simulink model "Sim_Metabolico_ParamE2"  (R2024b)
settings: Solver=ode15s  StartTime=0.0  StopTime=30  RelTol=1e-12  AbsTol=1e-6  EnableMultiTasking=on
values from neighbouring files (symbols this model uses):
  k_I_sec = 10    [Fig10_ParametricAnalysis_kIsec_JTB.m]    (also in Fig11_ParametricAnalysis_kIupJTB.m; Fig12_ParametricAnalysis_kP4sec_JTB.m; SensitivityAnalysisFIM_JTBpaper.m)
  k_I_up = 12    [Fig10_ParametricAnalysis_kIsec_JTB.m]    (also in Fig11_ParametricAnalysis_kIupJTB.m; Fig12_ParametricAnalysis_kP4sec_JTB.m; SensitivityAnalysisFIM_JTBpaper.m = 11.999988)
settings Model: Creator=Usuario  LastModifiedBy=carolinaramirezmazo
settings SolverCC: AutoScaleAbsTol=off  AlgebraicLoopSolver=TrustRegion
settings DataIOCC: LimitDataPoints=on  SaveFormat=Array  ReturnWorkspaceOutputs=off
settings OptimizationCC: LifeSpan=inf
settings DebuggingCC: SolverPrmCheckMsg=warning  UnconnectedInputMsg=warning  UnconnectedOutputMsg=warning  UnconnectedLineMsg=warning  SFUnexpectedBacktrackingDiag=warning  SFNoUnconditionalDefaultTransitionDiag=warning  SFExecutionAtInitializationDiag=none  ArithmeticOperatorsInVariantConditions=warning
settings HardwareCC: ProdBitPerPointer=32  ProdBitPerSizeT=32  ProdBitPerPtrDiffT=32  ProdLargestAtomicFloat=None  ProdIntDivRoundTo=Undefined  ProdEndianess=Unspecified  ProdWordSize=32  ProdHWDeviceType=32-bit Generic
settings ModelReferenceCC: EnableRefExpFcnMdlSchedulingChecks=on  PropagateSignalLabelsOutOfModel=off
settings SFSimCC: SimUseLocalCustomCode=off  CustomCodeUndefinedFunction=UseInterfaceOnly
settings RTWCC: RTWUseLocalCustomCode=off  GPUComputeCapability=3.5  DLArmComputeVersion=19.05
settings CodeAppCC: StateflowObjectComments=on
settings GRTTargetCC: TargetLangStandard=C89/C90 (ANSI)
settings ConfigComp: CovMetricSettings=dw  CovSaveCumulativeToWorkspaceVar=on  CovSaveSingleToWorkspaceVar=on  CovExternalEMLEnable=off  CovSFcnEnable=off

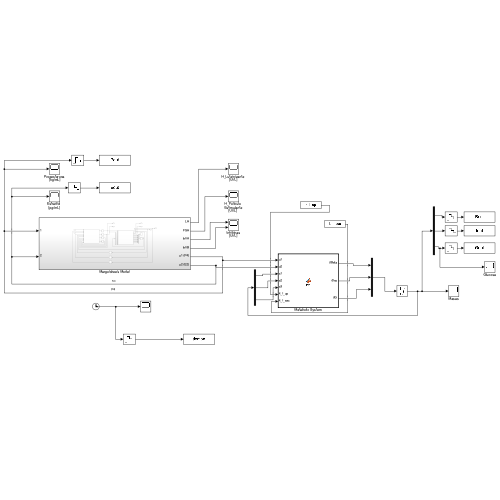
[thumbnail: Simulink's stored preview of the top-level diagram]
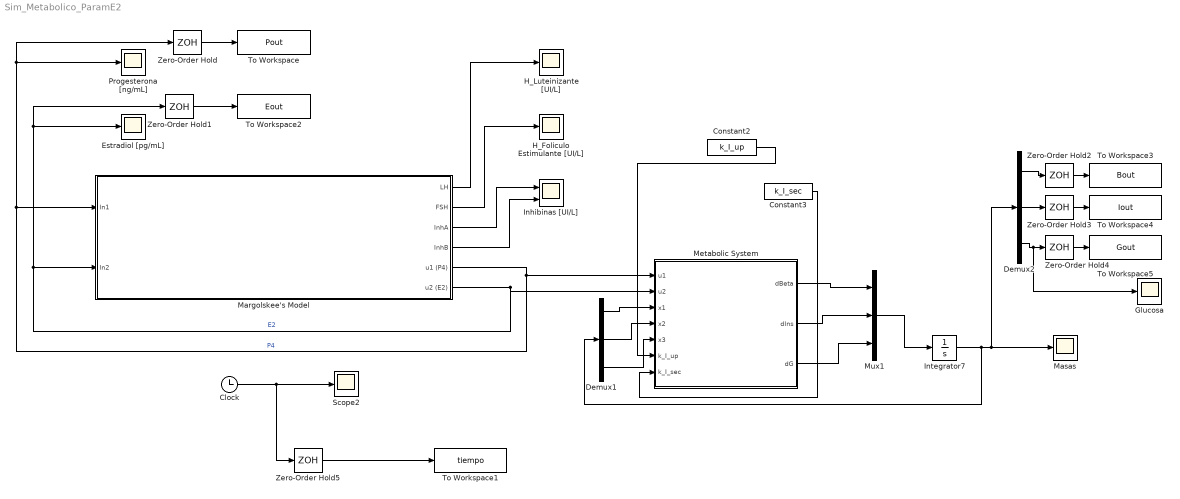
== system Sim_Metabolico_ParamE2 ==
  Clock : Clock
  Constant2 : Constant  Value=k_I_up
  Constant3 : Constant  Value=k_I_sec
  Demux1 : Demux  Outputs=3
  Demux2 : Demux  Outputs=3
  Estradiol [pg/mL] : Scope
  Glucosa : Scope
  "H_Foliculo Estimulante [UI/L] " : Scope
  H_Luteinizante [UI/L] : Scope
  Inhibinas [UI/L] : Scope  NumInputPorts=2
  Integrator7 : Integrator  InitialCondition=[850,7,108.1]  LimitOutput=on  LowerSaturationLimit=0
  Margolskee's Model : Subsystem
  Masas : Scope
  Metabolic System : MATLAB Function  TreatAsAtomicUnit=on
  Mux1 : Mux  Inputs=3
  Progesterona [ng/mL] : Scope
  Scope2 : Scope
  To Workspace : ToWorkspace  VariableName=Pout  SampleTime=-1
  To Workspace1 : ToWorkspace  VariableName=tiempo  SampleTime=-1
  To Workspace2 : ToWorkspace  VariableName=Eout  SampleTime=-1
  To Workspace3 : ToWorkspace  VariableName=Bout  SampleTime=-1
  To Workspace4 : ToWorkspace  VariableName=Iout  SampleTime=-1
  To Workspace5 : ToWorkspace  VariableName=Gout  SampleTime=-1
  Zero-Order Hold{,1..5} (6 alike) : ZeroOrderHold  SampleTime=0.01
  wires:
  Demux1/1 -> Metabolic System/3(x1)
  Demux1/2 -> Metabolic System/4(x2)
  Demux1/3 -> Metabolic System/5(x3)
  Metabolic System/1(dBeta) -> Mux1/1
  Metabolic System/2(dIns) -> Mux1/2
  Metabolic System/3(dG) -> Mux1/3
  Mux1/1 -> Integrator7/1
  Integrator7/1 -> Demux2/1, Masas/1, Demux1/1
  Margolskee's Model/3(InhA) -> Inhibinas [UI/L]/1
  Margolskee's Model/1(LH) -> H_Luteinizante [UI/L]/1
  Margolskee's Model/4(InhB) -> Inhibinas [UI/L]/2
  Margolskee's Model/2(FSH) -> "H_Foliculo Estimulante [UI/L] "/1
  Margolskee's Model/5(u1 (P4)) -> Zero-Order Hold/1, Progesterona [ng/mL]/1, Margolskee's Model/1(In1), Metabolic System/1(u1)  "P4"
  Clock/1 -> Zero-Order Hold5/1, Scope2/1
  Margolskee's Model/6(u2 (E2)) -> Zero-Order Hold1/1, Estradiol [pg/mL]/1, Margolskee's Model/2(In2), Metabolic System/2(u2)  "E2"
  Zero-Order Hold/1 -> To Workspace/1
  Zero-Order Hold1/1 -> To Workspace2/1
  Zero-Order Hold2/1 -> To Workspace3/1
  Zero-Order Hold3/1 -> To Workspace4/1
  Zero-Order Hold4/1 -> To Workspace5/1
  Demux2/2 -> Zero-Order Hold3/1
  Demux2/1 -> Zero-Order Hold2/1
  Demux2/3 -> Glucosa/1, Zero-Order Hold4/1
  Zero-Order Hold5/1 -> To Workspace1/1
  Constant2/1 -> Metabolic System/6(k_I_up)
  Constant3/1 -> Metabolic System/7(k_I_sec)

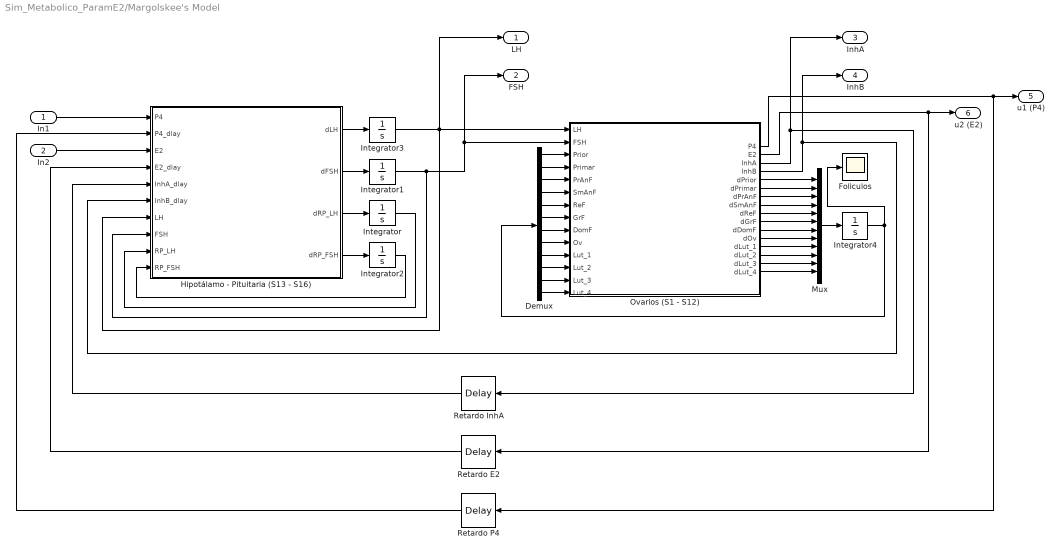
== system Sim_Metabolico_ParamE2/Margolskee's Model ==
  In1 : Inport
  In2 : Inport  Port=2
  Demux : Demux  Outputs=12
  Foliculos : Scope
  Hipotálamo - Pituitaria (S13 - S16) : MATLAB Function  TreatAsAtomicUnit=on
  Integrator : Integrator  InitialCondition=78.5  LimitOutput=on  LowerSaturationLimit=0
  Integrator1 : Integrator  InitialCondition=11  LimitOutput=on  LowerSaturationLimit=0
  Integrator2 : Integrator  InitialCondition=12  LimitOutput=on  LowerSaturationLimit=0
  Integrator3 : Integrator  InitialCondition=9.05  LimitOutput=on  LowerSaturationLimit=0
  Integrator4 : Integrator  InitialCondition=[265000, 100, 1.15, 3.98, 40.4, 53.1, 23.3, 16.0, 91.3, 320, 438, 362]  LimitOutput=on  LowerSaturationLimit=0
  Mux : Mux  Inputs=12
  Ovarios (S1 - S12) : MATLAB Function  TreatAsAtomicUnit=on
  Retardo E2 : TransportDelay  DelayTime=0.187
  Retardo InhA : TransportDelay  DelayTime=1.38
  Retardo P4 : TransportDelay  DelayTime=2
  LH : Outport  VectorParamsAs1DForOutWhenUnconnected=off
  FSH : Outport  Port=2  VectorParamsAs1DForOutWhenUnconnected=off
  InhA : Outport  Port=3  VectorParamsAs1DForOutWhenUnconnected=off
  InhB : Outport  Port=4  VectorParamsAs1DForOutWhenUnconnected=off
  u1 (P4) : Outport  Port=5  VectorParamsAs1DForOutWhenUnconnected=off
  u2 (E2) : Outport  Port=6  VectorParamsAs1DForOutWhenUnconnected=off
  wires:
  Mux/1 -> Integrator4/1
  Integrator3/1 -> LH/1, Hipotálamo - Pituitaria (S13 - S16)/7(LH), Ovarios (S1 - S12)/1(LH)
  Ovarios (S1 - S12)/3(InhA) -> InhA/1, Retardo InhA/1
  Demux/4 -> Ovarios (S1 - S12)/6(SmAnF)
  Hipotálamo - Pituitaria (S13 - S16)/1(dLH) -> Integrator3/1
  Integrator/1 -> Hipotálamo - Pituitaria (S13 - S16)/9(RP_LH)
  Demux/12 -> Ovarios (S1 - S12)/14(Lut_4)
  Demux/1 -> Ovarios (S1 - S12)/3(Prior)
  Ovarios (S1 - S12)/15(dLut_3) -> Mux/11
  Retardo InhA/1 -> Hipotálamo - Pituitaria (S13 - S16)/5(InhA_dlay)
  Demux/3 -> Ovarios (S1 - S12)/5(PrAnF)
  Hipotálamo - Pituitaria (S13 - S16)/2(dFSH) -> Integrator1/1
  Retardo P4/1 -> Hipotálamo - Pituitaria (S13 - S16)/2(P4_dlay)
  Ovarios (S1 - S12)/4(InhB) -> Hipotálamo - Pituitaria (S13 - S16)/6(InhB_dlay), InhB/1
  Integrator1/1 -> Hipotálamo - Pituitaria (S13 - S16)/8(FSH), Ovarios (S1 - S12)/2(FSH), FSH/1
  In2/1 -> Hipotálamo - Pituitaria (S13 - S16)/3(E2)
  Ovarios (S1 - S12)/9(dReF) -> Mux/5
  Integrator4/1 -> Demux/1, Foliculos/1
  Ovarios (S1 - S12)/12(dOv) -> Mux/8
  Integrator2/1 -> Hipotálamo - Pituitaria (S13 - S16)/10(RP_FSH)
  Demux/2 -> Ovarios (S1 - S12)/4(Primar)
  Ovarios (S1 - S12)/2(E2) -> Retardo E2/1, u2 (E2)/1
  Ovarios (S1 - S12)/10(dGrF) -> Mux/6
  Ovarios (S1 - S12)/16(dLut_4) -> Mux/12
  Ovarios (S1 - S12)/6(dPrimar) -> Mux/2
  Ovarios (S1 - S12)/5(dPrior) -> Mux/1
  Demux/7 -> Ovarios (S1 - S12)/9(DomF)
  Ovarios (S1 - S12)/7(dPrAnF) -> Mux/3
  Demux/6 -> Ovarios (S1 - S12)/8(GrF)
  Hipotálamo - Pituitaria (S13 - S16)/3(dRP_LH) -> Integrator/1
  Ovarios (S1 - S12)/11(dDomF) -> Mux/7
  Demux/11 -> Ovarios (S1 - S12)/13(Lut_3)
  Ovarios (S1 - S12)/8(dSmAnF) -> Mux/4
  Demux/5 -> Ovarios (S1 - S12)/7(ReF)
  Ovarios (S1 - S12)/13(dLut_1) -> Mux/9
  Demux/8 -> Ovarios (S1 - S12)/10(Ov)
  Ovarios (S1 - S12)/14(dLut_2) -> Mux/10
  Demux/10 -> Ovarios (S1 - S12)/12(Lut_2)
  Demux/9 -> Ovarios (S1 - S12)/11(Lut_1)
  Retardo E2/1 -> Hipotálamo - Pituitaria (S13 - S16)/4(E2_dlay)
  Hipotálamo - Pituitaria (S13 - S16)/4(dRP_FSH) -> Integrator2/1
  Ovarios (S1 - S12)/1(P4) -> Retardo P4/1, u1 (P4)/1
  In1/1 -> Hipotálamo - Pituitaria (S13 - S16)/1(P4)

== matlab function Sim_Metabolico_ParamE2/Margolskee's Model/Ovarios (S1 - S12) ==
  data: P4 output; E2 output; InhA output; InhB output; dPrior output; dPrimar output; dPrAnF output; dSmAnF output; LH input; FSH input; Prior input; Primar input; PrAnF input; SmAnF input; ReF input; GrF input; DomF input; Ov input; dReF output; dGrF output; dDomF output; dOv output; Lut_1 input; Lut_2 input; Lut_3 input; Lut_4 input; dLut_1 output; dLut_2 output; dLut_3 output; dLut_4 output
function [P4,E2,InhA,InhB,dPrior,dPrimar,dPrAnF,dSmAnF,dReF,dGrF,dDomF,dOv,...
    dLut_1,dLut_2,dLut_3,dLut_4]= ...
    fcn(LH,FSH,Prior,Primar,PrAnF,SmAnF,ReF,GrF,DomF,Ov,Lut_1,Lut_2,Lut_3,Lut_4)
%% Modelo de Ovarios 
% El modelo representa diferentes etapas de los oocitos que incluye desgaste  
% del número de folículos, el cual esta límitado desde el nacimiento. 

% Las entradas son las concentraciones sistemicas de hormonas Luteinizante (LH),
% y Foliculo Estimulante (FSH) generadas en la pituitaria. 

% Las salidas son las hormonas Progesterona (P4), Estradiol (E2), Inhibina (Inh)
% y Antimulleriana (AMH). Esta ultima tiene una acción feedback sobre el sistema

%% Nomenclatura de los sistemas ===========================================
% S1 = Prior = Folículo primordial
% S2 = Primar = Folículo primario 
% S3 = PrAnF = Folículos preantales
% S4 = SmAnF = Folículos antrales pequeños 
% S5 = ReF = Folículos reclutados
% S6 = GrF = Folículos en crecimiento
% S7 = DomF = Folículo dominante 
% S8 = Ov = Folículo ovulatorio 
% S9 = Lut_1 = Cuerpo luteo fase 1
% S10 = Lut_2 = Cuerpo luteo fase 2
% S11 = Lut_3 = Cuerpo luteo fase3
% S12 = Lut_4 = Cuerpo luteo fase 4

%% Parametros =============================================================
% Parametros Sistemas S1 y S2 (Revisado)
c_AMH = 0.226;      % [mL/ng]
c_prm = 1.37E-5;    % [1/fóliculo] (Candidato)
r_surv = 0.014;     % [~]
r_1 = 0.00102;      % [1/dia]
r_2 = 0.00694;      % [1/dia]

% Parametros Sistemas S3 y S12 (Revisados)
vol_2 = 0.500;      % [mm^3]
Km_f1 = 9.82;       % [UI/L]
Km_f2 = 10.4;       % [UI/L]
Km_f3 = 5.08;       % [UI/L]
Ki_AMH = 20.7;      % [ng/mL]
r_3 = 0.759;        % [1/dia]
r_4 = 2.23;         % [L/(dia*UI)]
r_5 = 1.21;         % [1/dia]
c_1 = 0.918;        % [1/dia]
c_2 = 0.0575;       % [(L/IU)^delta/dia]
c_3 = 0.0241;       % [L/(IU*dia)]
c_4 = 0.0307;       % [L/(IU*dia)]
c_5 = 0.198;        % [(L/IU)^gamma/dia]
c_6 = 0.00519;      % [L/(IU*dia)]
c_7 = 0.686;        % [dia]
k_1 = 0.416;        % [1/dia]
k_2 = 0.405;        % [1/dia]   
k_3 = 0.551;        % [1/dia]
k_4 = 0.903;        % [1/dia]

% Parametros de cinéticas de Hill (Revisados)
alfa = 29.1;        % [~]
beta = 2.06;        % [~]
gamma = 2.95;       % [~]
delta = 0.999;      % [~]
omega = 0.363;      % [~]

% Parámetros ecuaciones algebraicas (Revisados)
e_0 = 30;           % [pg/mL]
e_1 = 0.04;         % [pg/(mL*mm^3)]
e_2 = 0.065;        % [pg/(mL*mm^3)]
e_3 = 0.1;          % [pg/(mL*mm^3)]
p_0 = 0;            % [ng/(mL*mm^3)]
p_1 = 0.0085;       % [ng/(mL*mm^3)]
p_2 = 0;            % [ng/(mL*mm^3)]
h_0 = 0;            % [IU/mL]
h_1 = 0.0035;       % [IU/(mL*mm^3)]
h_2 = 0.0021;       % [IU/(mL*mm^3)]
h_3 = 0.0021;       % [IU/(mL*mm^3)]
j_0 = 15;           % [IU/mL]
j_1 = 20.2;         % [pg/(mL*mm^3)]
j_2 = 0.0138;       % [pg/(mL*mm^3)]
a_1 = 0.0437;       % [ng/(mL*folículo)]
a_2 = 0;            % [~]
a_3 = 0;            % [~]

%% Ecuaciones algebraicas (Hormonas) ====================================== (Revisado)
E2 = e_0 + (e_1*GrF) + (e_2*DomF) + (e_3*Lut_4);
P4 = p_0 + (p_1*Lut_3) + (p_2*Lut_4);
InhA = h_0 + (h_1*DomF) + (h_2*Lut_2) + (h_3*Lut_3);
InhB = j_0 + (j_1*SmAnF) + (j_2*Ov);
AMH = (a_1*Primar) + (a_2*PrAnF) + (a_3*SmAnF);

%% Ecuaciones diferenciales (Folículos) =================================== (Revisado)
dPrior = -(r_1*Prior)/(1 + c_prm*Prior + c_AMH*AMH);
dPrimar = ((r_surv*r_1*Prior)/(1 + c_prm*Prior + c_AMH*AMH)) - (r_2*Primar);
dPrAnF = (vol_2*r_2*Primar) - ((r_3*PrAnF*(FSH^alfa))/((Km_f1^alfa)+(FSH^alfa)));
dSmAnF = ((r_3*PrAnF*(FSH^alfa))/((Km_f1^alfa)+(FSH^alfa))) +...
    (((r_4*(FSH^beta))/((Km_f2^beta)+(FSH^beta))) - r_5)*SmAnF;
dReF = (r_5*SmAnF) + (((c_1*(FSH^gamma))/((Km_f3^gamma)+(FSH^gamma))) - (c_2*(LH^delta)))*ReF;
dGrF = (c_2*(LH^delta)*ReF) + (((c_3*FSH)/(1+(AMH/Ki_AMH)))-(c_4*LH))*GrF;
dDomF = (c_4*LH*GrF) - (c_5*(LH^omega)*DomF);
dOv = (c_5*(LH^omega)*DomF) + (c_6*LH*Ov) - (c_7*Ov);
dLut_1 = (c_7*Ov) - (k_1*Lut_1);
dLut_2 = (k_1*Lut_1) - (k_2*Lut_2);
dLut_3 = (k_2*Lut_2) - (k_3*Lut_3);
dLut_4 = (k_3*Lut_3) - (k_4*Lut_4);

== matlab function Sim_Metabolico_ParamE2/Margolskee's Model/Hipotálamo - Pituitaria (S13 - S16) ==
  data: dLH output; dFSH output; P4 input; P4_dlay input; dRP_LH output; dRP_FSH output; E2 input; E2_dlay input; InhA_dlay input; InhB_dlay input; LH input; FSH input; RP_LH input; RP_FSH input
function [dLH, dFSH, dRP_LH, dRP_FSH] = ...
    fcn(P4, P4_dlay, E2, E2_dlay, InhA_dlay, InhB_dlay, LH, FSH, RP_LH, RP_FSH)
%% Modelo del Hipotálamo y la pituitaria
% El modelo representa la producción de hormonas que controlan la
% maduración de los oocitos en los ovarios. 

% Las entradas son las concentraciones sistemicas de Progesterona (P4),
% Estradiol (E2) e Inhibina A y B (InhA) (InhB) generadas en los ovarios. 

% Las salidas son las hormonas Luteinizante (LH) y Foliculo Estimulante (FSH)

%% Nomenclatura de los sistemas ===========================================
% S13 = RP_LH = hormona luteinizante en pituitaria
% S14 = LH = hormona luteinizante en sangre
% S15 = RP_FSH = foliculo estimulante en pituitaria
% S16 = FSH = foliculo estimulante en sangre

%% Parametros ============================================================= (Revisados)
V_0LH = 343;        % [IU/day]
V_1LH = 8110;       % [IU/day]
Km_LH = 247;        % [pg/mL]
Ki_LH_P = 155;      % [ng/mL]
k_LH = 1.01;        % [1/day]
cl_LH = 14;         % [1/day]
c_LH_P = 1.10;      % [mL/ng]
c_LH_E = 0.00398;   % [mL/ng]

V_FSH = 616;        % [IU/day]
Ki_FSH_InhA = 2.58; % [IU/mL]
Ki_FSH_InhB = 120;  % [pg/mL]
k_FSH = 1.04;       % [1/day]
cl_FSH = 8.21;      % [1/day]
c_FSH_P = 130;      % [mL/ng]
c_FSH_E = 0.00525;  % [mL^2/pg^2]

v = 2.5;            % [L]

%% Ecuaciones diferenciales =============================================== (Revisado)
dRP_LH = ((V_0LH + ((V_1LH*(E2_dlay^8))/((Km_LH^8)+(E2_dlay^8))))/(1+(P4_dlay/Ki_LH_P))) -...
    ((k_LH*RP_LH*(1+c_LH_P*P4))/(1+c_LH_E*E2));

dLH = ((1/v)*((k_LH*RP_LH*(1+c_LH_P*P4))/(1+c_LH_E*E2))) - (cl_LH*LH);

dRP_FSH = (V_FSH/(1+(InhA_dlay/Ki_FSH_InhA)+(InhB_dlay/Ki_FSH_InhB))) -...
    ((k_FSH*RP_FSH*(1+c_FSH_P*P4))/(1+(c_FSH_E*(E2^2))));

dFSH = ((1/v)*((k_FSH*RP_FSH*(1+c_FSH_P*P4))/(1+(c_FSH_E*(E2^2))))) - (cl_FSH*FSH);

== matlab function Sim_Metabolico_ParamE2/Metabolic System ==
  data: dBeta output; u1 input; u2 input; x1 input; x2 input; x3 input; dIns output; dG output; k_I_up input; k_I_sec input
function [dBeta,dIns,dG]  =  fcn(u1,u2,x1,x2,x3,k_I_up,k_I_sec)


%% State Variables
Beta=x1;
Ins=x2;
G=x3;
Ue=u2;
Up=u1;

%Parameters & Differential equations=============
R_0= 890; %890Non Fasting 864Fasting       %[mg/dL.d]  %Net rate of production from Topp -fasting
E_G0=8; %8 Non fasting 10 Fasting [1.d]       %Insulin independent glucose disposal rate-Total glucose effectiveness at "zero insulin" Taken from Topp
k_cl=432; %[1/d]       %Insulin clearance rate. Taken from Topp
%k_I_sec=10; %%[µU/mL.d.mg] maximum rate of Insulin secretion/mg
K_G_sec=100;  %[mg/dL]Glucose threshold to trigger Insulin secretion
Ks_E2=62; % E2 threshold to trigger Insulin sensitivity stimulatory effect
K_E2_sec=33; % E2 threshold to trigger Insulin secretion stimulatory effect;

%===========Insulin Kinetics==============================
Prom_sec=Ue/((K_E2_sec+Ue)); %2
%k_P4_sec=0.3/(16.7^1.5); %0.004395887283525: 0.004 in the table

%% P4 inhibiting also I secretion: makes the glucose pretty much constrant-square during lutheal 
 Ins_sec=k_I_sec.*Prom_sec.*(G)/(K_G_sec+G); %[µU/mg.d]

 %% =============Beta Dynamics Parameters========================
%From literature:
%apoptosis rate 5% Apoptosis in pancreatic β-islet cells in Type 2 diabetes Tatsuo Tomita
%In the human pancreas, β-cell mass has been reported to vary from 0.6 to 2.1 g, and the 
%amount of insulin in the gland has been observed to range from 50 to 250 ug/g (Marchetti and Ferrannini,2015)

%The  frequency  of  β-cell  replication  was  very  low  at  0.04-0.06%  of  β-cell  mass
k_beta=0.00045;   %0.0355 0.0343 0.0335 IFAC =0.03069 0.00033 0.00046 0.0003 0.00013 %mgmL/pg.d maximum growth rate with apop 0.5% and Ks 1500
K_beta_G_Apop=125;%150 ifac
K_beta_G_g=70;%70
K_beta_E2=50;

%Replication  and  apoptosis  rate  should  be  about  the  same  to  maintain  the  β-cell  mass  at  a  delicate  balance
%http://dx.doi.org/10.17305/bjbms.2016.919-Tatsuo Tomita*
%mu_Beta_Apop=0.0146; %0.0086 0.00833 0.013 0.016 0.0013 0.005 0.1 1.6; 
k_beta_Apop=0.0004;

%==============Beta  Kinetics=============================
mu_beta_growth=k_beta*(Ue/(K_beta_E2+Ue))*G/(K_beta_G_g+G);

mu_Beta_Apop=k_beta_Apop*G/(K_beta_G_Apop+G);

%% Insulin dependent glucose uptake,as a function of Estradiol
%k_I_up=12; % 6.5 9 4.5IFAC 6 4 16 2e2[mL/pg.d] very sensitive with 2 monod 1.1e+2 shape maximum rate of Insulin reception matching with S_I in literature (for glucose uptake)
Ks_up=70; % 6.5 4 15 with kgrowth 0.03 and iup 1.6
%% two Monods
  Prom=Ue/(Ks_E2+Ue);

  SI=k_I_up*Prom*1/(Ks_up+Ins);
  
%% Two monods multipliyng promoting and inhib
Ins_up=SI*Ins;

%=========Edos - Estructura básica =========================
dBeta=(Beta*mu_beta_growth-Beta*mu_Beta_Apop);
dIns=(Beta*Ins_sec)-(k_cl*Ins); 
dG=R_0-((E_G0+(Ins_up))*G);
